simulink model "cinematica_fcn_block"  (R2018a)
settings: Solver=VariableStepAuto  StartTime=0.0  StopTime=10.0  RelTol=1e-3
settings Model: Creator=LabT5  LastModifiedBy=LabT5

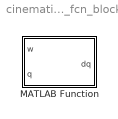
== system cinematica_fcn_block ==
  MATLAB Function : MATLAB Function  TreatAsAtomicUnit=on

== matlab function cinematica_fcn_block/MATLAB Function ==
  data: w input; dq output; q input
function dq = cinematica(w,q)
%#eml
wx = w(1);
wy = w(2);
wz = w(3);

q = q/norm(q);
qteta = q(1);
qx = q(2);
qy = q(3);
qz = q(4);

W = [0 -wx -wy -wz; wx 0 wz -wy; wy -wz 0 wx; wz wy -wx 0];
dq=0.5*W*[qteta qx qy qz]';
